simulink model "LTE_simulationslx"  (R2019a)
settings: Solver=ode45  StartTime=0.0  StopTime=0.003  RelTol=1e-3  EnableMultiTasking=on
undefined symbols (not defined in the file or in its folder): doppler, Iter, Len, Max, Variance
libraries: dspobslib x6, commsequence2 x6, commblkintrlv2 x6, dspindex x5, commcnvcod2 x4, commchan3 x2, commcrc2 x2, commdigbbndam3 x2, dspxfrm3 x2, commseqgen2 x2, commutil2 x2, commrandsrc3 x1
settings Model: Creator=Natalia  LastModifiedBy=Bill
settings DataIOCC: LimitDataPoints=on  SaveFormat=Array  SignalLoggingSaveFormat=ModelDataLogs  ReturnWorkspaceOutputs=off
settings OptimizationCC: ExpressionDepthLimit=2147483647  LifeSpan=inf
settings DebuggingCC: UnderspecifiedInitializationDetection=Classic  MergeDetectMultiDrivingBlocksExec=none  SolverPrmCheckMsg=warning  FcnCallInpInsideContextMsg=warning  StateNameClashWarn=warning  SFUnexpectedBacktrackingDiag=warning  SFNoUnconditionalDefaultTransitionDiag=warning  SFExecutionAtInitializationDiag=none  ArithmeticOperatorsInVariantConditions=warning
settings HardwareCC: ProdBitPerPointer=32  ProdBitPerSizeT=32  ProdBitPerPtrDiffT=32  ProdLargestAtomicFloat=None  ProdIntDivRoundTo=Undefined  ProdEndianess=Unspecified  ProdWordSize=32  ProdHWDeviceType=32-bit Generic
settings ModelReferenceCC: PropagateSignalLabelsOutOfModel=off
settings SFSimCC: SimUseLocalCustomCode=off  SimParseCustomCode=off
settings RTWCC: RTWUseLocalCustomCode=off
settings CodeAppCC: StateflowObjectComments=on
settings GRTTargetCC: TargetLangStandard=C89/C90 (ANSI)  GeneratePreprocessorConditionals=Disable all  CombineOutputUpdateFcns=off  GRTInterface=on
settings ConfigComp: CovMetricSettings=dw  CovHtmlReporting=on  CovSaveCumulativeToWorkspaceVar=on  CovSaveSingleToWorkspaceVar=on  CovExternalEMLEnable=off

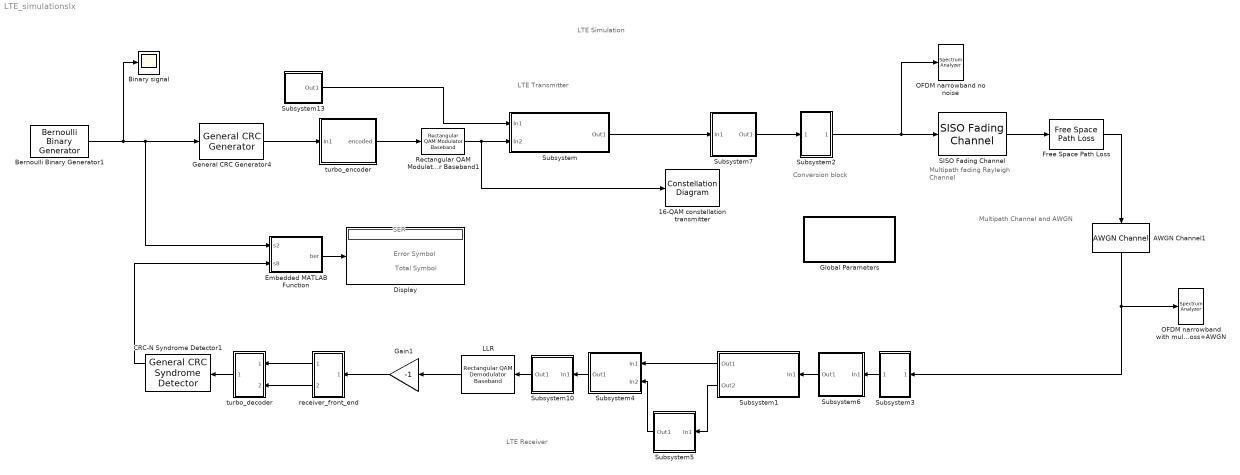
== system LTE_simulationslx ==
  note: SER
  note: Error Symbol
  note: Total Symbol
  note: LTE Simulation
  note: LTE Transmitter
  note: LTE Receiver
  note: Multipath Channel
      | and AWGN
  note: Conversion block
  note: Multipath fading Rayleigh Channel
  16-QAM constellation transmitter : ConstellationDiagram  Tag=ScatterPlot
  AWGN Channel1 : commchan3/AWGN Channel  InputProcessing=Columns as channels (frame based)  seed=32965  noiseMode="Signal to noise ratio  (Eb/No)"  EbNodB=12  EsNodB=1  SNRdB=2  bitsPerSym=1  Ps=30/(5.5e5*11/15*2.4)*1.08  Tsym=80e-6  variance=1
      settings: SourceProductName=Communications Toolbox
  Bernoulli Binary Generator1 : commrandsrc3/Bernoulli Binary Generator  ProbabilityOfZero=.5  SeedSource=Auto  Seed=0  SampleTime=1  SamplesPerFrame=20  OutputDataType=boolean  SimulateUsing=Code generation
      settings: SourceProductName=Communications Toolbox
  Binary signal : Scope
  CRC-N Syndrome Detector1 : commcrc2/General CRC Syndrome Detector  genPoly=[1 1 0 0 0 0 0 0 0 0 1 0 1 0 0 0 1 0 0 0 0 0 0 0 1]  iniStates=[0]  directMethod=off  reflectInputBytes=off  reflectChecksums=off  finalXOR=0  numChecksums=1
      settings: SourceProductName=Communications Toolbox  SourceProductBaseCode=CM
  Display : Display
  Embedded MATLAB Function : MATLAB Function  TreatAsAtomicUnit=on
  Free Space Path Loss : commrflib2/Free Space Path Loss  mode=Decibels  dB=10  d=0.100  fc=1920
      settings: SourceProductName=Communications Toolbox  SourceProductBaseCode=CM
  Gain1 : Gain  Gain=-1  SaturateOnIntegerOverflow=on  OutDataTypeStr=Inherit: Same as input  ParamDataTypeStr=Inherit: Same as input
  General CRC Generator4 : commcrc2/General CRC Generator  genPoly=[24,23,18,17,14,11,10,7,6,5,1,0]  iniStates=[0]  directMethod=off  reflectInputBytes=off  reflectChecksums=off  finalXOR=0  numChecksums=1
      settings: SourceProductName=Communications Toolbox  SourceProductBaseCode=CM
  Global Parameters : Subsystem  mask(Global Parameters){EbNodB=11, Len=44, Iter=5, Seed=54123}
      mask prompts: EbNodB "Eb/No in dB:"; Len "Block size:"; Iter "Number of iterations:"
      mask help: Load global parameters in MATLAB workspace.
      mask init:
      | turbo_code_punc_setup;
      mask Callback EbNodB: turbo_code_setup;
      mask Callback Len: turbo_code_setup
      mask Callback Iter: turbo_code_setup;
      mask Callback Seed: turbo_code_setup;
      mask Display: disp(['Eb/No ' num2str(EbNodB,'%3.1f') 'dB'  sprintf('\n') 'Block size   ' num2str(Len,'%7.0f')  sprintf('\n') 'Iterations   ' num2str(Iter,'%3.0f')   sprintf('\n') 'Seed   ' num2str(Seed,'%7.0f')])
  LLR : commdigbbndam3/Rectangular QAM Demodulator Baseband  M=16  OutType=Bit  DecType=Log-likelihood ratio  VarSource=Dialog  Variance=Variance  Dec=Gray  Mapping=[0:15]  PowType=Average Power  MinDist=2  AvgPow=0.5  PeakPow=1  Ph=0  outDtype1=double  outDtype2=double  derotateFactorWordLen=16  derotateFactorDataTypeStr=Inherit: Same word length as input  derotateFactorLastDataTypeStr=Inherit: Same word length as input  denormFactorWordLen=16  denormFactorDataTypeStr=Inherit: Same word length as input  denormFactorLastDataTypeStr=Inherit: Same word length as input  prodOutWordLen=32  prodOutOverflowMode=Wrap  prodOutRoundingMode=Floor  prodOutOvFlMode=off  prodOutOvFlModeLastStrValue=off  sumWordLen=32
      settings: SourceProductName=Communications Toolbox
  OFDM narrowband no noise : SpectrumAnalyzer
  OFDM narrowband with multipath fading +pathloss+AWGN : SpectrumAnalyzer
  Rectangular QAM Modulator Baseband1 : commdigbbndam3/Rectangular QAM Modulator Baseband  M=16  InType=Bit  Enc=Gray  Mapping=[0:15]  PowType=Average Power  MinDist=2  AvgPow=0.5  PeakPow=1  Ph=0  outDtype=double  outWordLen=16  outUDDataType=sfix(16)  outFracLenMode=Best precision  outFracLen=15  outDataTypeStr=double  outLastDataTypeStr=double
      settings: SourceProductName=Communications Toolbox
  SISO Fading Channel : commchan3/SISO Fading Channel  InheritSampleRate=on  SampleRate=1  PathDelays=[0 2e-6]  AveragePathGains=[0 -3]  NormalizePathGains=on  FadingDistribution=Rayleigh  KFactor=3  DirectPathDopplerShift=0  DirectPathInitialPhase=0  MaximumDopplerShift=40  DopplerSpectrum=doppler('Jakes')  ChannelInterpolationMethod=Polyphase  RandomStream=mt19937ar with seed  RandomNumGenerator=mt19937ar  Seed=73  PathGainsOutputPort=off  ChannelFilterDelayOutputPort=off  SimulateUsing=Interpreted execution  Visualization=Off  PathsForDopplerDisplay=1  SamplesToDisplay=25%
      settings: SourceProductName=Communications Toolbox
  Subsystem : Subsystem
      mask Display: disp('OFDM Baseband\nModulator\ndan\nAdd Cyclic Prefix')
  Subsystem1 : Subsystem
      mask Display: disp('OFDM Baseband\nDemodulator\ndan \nRemove Cyclic prefix')
  Subsystem10 : Subsystem
      mask Display: disp('Remove\nZero')
  Subsystem13 : Subsystem
      mask Display: disp('Training')
  Subsystem2 : Subsystem  Tag=Conversion block
      mask Display: disp('P/S')
  Subsystem3 : Subsystem
      mask Display: disp('S/P')
  Subsystem4 : Subsystem
      mask Display: disp('Channel\nCompensation')
  Subsystem5 : Subsystem
      mask Display: disp('Channel\nEstimator')
  Subsystem6 : Subsystem
      mask Display: disp('Training\nSeparation')
  Subsystem7 : Subsystem
      mask Display: disp('Training\nInsertion')
  receiver_front_end : Subsystem
  turbo_decoder : Subsystem
  turbo_encoder : Subsystem
  wires:
  receiver_front_end/1(Out1) -> turbo_decoder/1(In1)
  receiver_front_end/2(Out2) -> turbo_decoder/2(In2)
  turbo_encoder/1(encoded) -> Rectangular QAM Modulator Baseband1/1
  LLR/1 -> Gain1/1
  Gain1/1 -> receiver_front_end/1(In1)
  Subsystem13/1(Out1) -> Subsystem/1(In1)
  Subsystem/1(Out1) -> Subsystem7/1(In1)
  Subsystem7/1(Out1) -> Subsystem2/1(In1)
  Rectangular QAM Modulator Baseband1/1 -> 16-QAM constellation transmitter/1, Subsystem/2(In2)
  Subsystem1/1(Out1) -> Subsystem4/1(In1)
  Subsystem1/2(Out2) -> Subsystem5/1(In1)
  Subsystem5/1(Out1) -> Subsystem4/2(In2)
  Subsystem4/1(Out1) -> Subsystem10/1(In1)
  Subsystem6/1(Out1) -> Subsystem1/1(In1)
  Subsystem3/1(Out1) -> Subsystem6/1(In1)
  Subsystem10/1(Out1) -> LLR/1
  Subsystem2/1(Out1) -> OFDM narrowband no noise/1, SISO Fading Channel/1
  AWGN Channel1/1 -> OFDM narrowband with multipath fading +pathloss+AWGN/1, Subsystem3/1(In1)
  General CRC Generator4/1 -> turbo_encoder/1(In1)
  turbo_decoder/1(Out1) -> CRC-N Syndrome Detector1/1
  Embedded MATLAB Function/1(ber) -> Display/1
  CRC-N Syndrome Detector1/1 -> Embedded MATLAB Function/2(s8)
  Bernoulli Binary Generator1/1 -> Binary signal/1, Embedded MATLAB Function/1(s2), General CRC Generator4/1
  Free Space Path Loss/1 -> AWGN Channel1/1
  SISO Fading Channel/1 -> Free Space Path Loss/1

== system LTE_simulationslx/Global Parameters ==

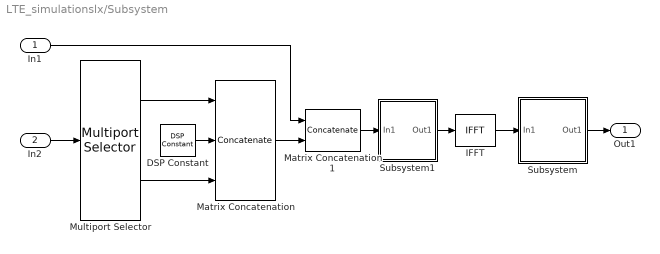
== system LTE_simulationslx/Subsystem ==
  In1 : Inport
  In2 : Inport  Port=2
  DSP Constant : dspobslib/DSP Constant  Value=0  SampleMode=Discrete  discreteOutput=Frame-based  continuousOutput=Sample-based  sampTime=16e-5/2  framePeriod=16e-5/2  dataType=Inherit from 'Constant value'  isSigned=on  wordLen=16  udDataType=sfix(16)  fracBitsMode=Best precision  numFracBits=15  InterpretAs1D=off  Ts=16e-5/2  FramebasedOutput=on
      settings: SourceProductName=DSP System Toolbox  SourceProductBaseCode=DS
  IFFT : dspxfrm3/IFFT  FFTImplementation=Auto  CompMethod=Table lookup  TableOpt=HYBRID  TableOptActive=Speed  BitRevOrder=off  cs_in=off  Normalize=on  InheritFFTLength=on  FFTLength=64  WrapInput=on  mode=Real  outSamplingMode=Frame based  roundingMode=Floor  overflowMode=off  firstCoeffDataTypeStr=Inherit: Same word length as input  firstCoeffLastDataTypeStr=Inherit: Same word length as input  outputMin=[]  outputMax=[]
      settings: SourceProductName=DSP System Toolbox
  Matrix Concatenation : Concatenate  NumInputs=3  Mode=Multidimensional array
  Matrix Concatenation1 : Concatenate  Mode=Multidimensional array  ConcatenateDimension=2
  Multiport Selector : dspindex/Multiport Selector  rowsOrCols=Rows  idxCellArray={1:11,12:22}  idxErrMode=Clip Index
  Subsystem : Subsystem
      mask Display: disp('Add\nCyclic Prefix')
  Subsystem1 : Subsystem
      mask Display: disp('Zero Pad')
  Out1 : Outport
  wires:
  IFFT/1 -> Subsystem/1(In1)
  Multiport Selector/1 -> Matrix Concatenation/1
  Multiport Selector/2 -> Matrix Concatenation/3
  DSP Constant/1 -> Matrix Concatenation/2
  Subsystem1/1(Out1) -> IFFT/1
  Subsystem/1(Out1) -> Out1/1
  In2/1 -> Multiport Selector/1
  Matrix Concatenation1/1 -> Subsystem1/1(In1)
  Matrix Concatenation/1 -> Matrix Concatenation1/2
  In1/1 -> Matrix Concatenation1/1

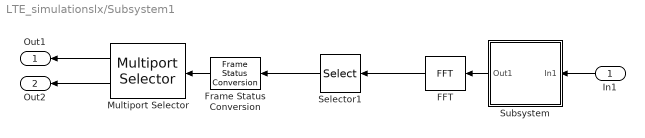
== system LTE_simulationslx/Subsystem1 ==
  In1 : Inport
  FFT : dspxfrm3/FFT  FFTImplementation=Auto  CompMethod=Table lookup  TableOpt=HYBRID  TableOptActive=Speed  BitRevOrder=off  Normalize=on  InheritFFTLength=on  FFTLength=64  WrapInput=on  roundingMode=Floor  overflowMode=off  firstCoeffDataTypeStr=Inherit: Same word length as input  firstCoeffLastDataTypeStr=Inherit: Same word length as input  outputMin=[]  outputMax=[]
  Frame Status Conversion : dspobslib/Frame Status Conversion  growRefPort=off  outframe=Frame-based
      settings: SourceProductName=DSP System Toolbox  SourceProductBaseCode=DS
  Multiport Selector : dspindex/Multiport Selector  rowsOrCols=Columns  idxCellArray={1,2}  idxErrMode=Clip Index
  Selector1 : Selector  NumberOfDimensions=2  InputPortWidth=64  IndexOptions=Index vector (dialog),Select all  Indices=[54:64,1:12],-1  OutputSizes=1
  Subsystem : Subsystem
      mask Display: disp('Remove\nCyclic Prefix')
  Out1 : Outport
  Out2 : Outport  Port=2
  wires:
  FFT/1 -> Selector1/1
  Selector1/1 -> Frame Status Conversion/1
  Subsystem/1(Out1) -> FFT/1
  In1/1 -> Subsystem/1(In1)
  Frame Status Conversion/1 -> Multiport Selector/1
  Multiport Selector/1 -> Out1/1
  Multiport Selector/2 -> Out2/1

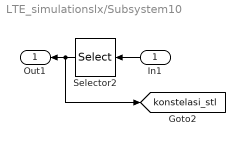
== system LTE_simulationslx/Subsystem10 ==
  In1 : Inport
  Selector2 : Selector  NumberOfDimensions=2  InputPortWidth=31  IndexOptions=Index vector (dialog),Select all  Indices=[1:11,13:23],-1  OutputSizes=1
  Out1 : Outport
  tag scope: konstelasi_stl=global
  wires:
  Selector2/1 -> Out1/1, [konstelasi_stl]
  In1/1 -> Selector2/1

== system LTE_simulationslx/Subsystem13 ==
  PN Sequence Generator : commseqgen2/PN Sequence Generator  poly=[1 0 0 0 0 1 1]  ini_sta=[0 0 0 0 0 1]  outBitMaskSource=Dialog parameter  shift=0  outVarSiz=off  maxOutSizeMode=Dialog parameter  maxOutSize=[10 1]  Ts=16e-5/2/23  frameBased=on  sampPerFrame=23  reset=off  bitPackedOutputs=off  outDataType=double  numPackedBits=8  bitPackDataSigned=off  bitPackedOutDType=double
      settings: SourceProductName=Communications Toolbox  SourceProductBaseCode=CM
  Unipolar to Bipolar Converter : commutil2/Unipolar to Bipolar Converter  M=2  polarity=Positive  dataType=Inherit via internal rule
      settings: SourceProductName=Communications Toolbox
  Out1 : Outport
  wires:
  PN Sequence Generator/1 -> Unipolar to Bipolar Converter/1
  Unipolar to Bipolar Converter/1 -> Out1/1

== system LTE_simulationslx/Subsystem2 ==
  In1 : Inport
  Unbuffer3 : Unbuffer
  Out1 : Outport
  wires:
  In1/1 -> Unbuffer3/1
  Unbuffer3/1 -> Out1/1

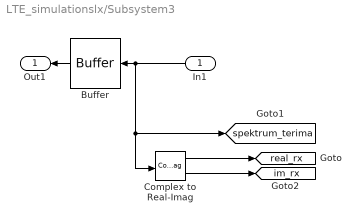
== system LTE_simulationslx/Subsystem3 ==
  In1 : Inport
  Buffer : Buffer  N=180
  Complex to Real-Imag : ComplexToRealImag
  Out1 : Outport
  tag scope: im_rx=global, real_rx=global, spektrum_terima=global
  wires:
  In1/1 -> Buffer/1, [spektrum_terima], Complex to Real-Imag/1
  Buffer/1 -> Out1/1
  Complex to Real-Imag/1 -> [real_rx]
  Complex to Real-Imag/2 -> [im_rx]

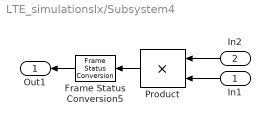
== system LTE_simulationslx/Subsystem4 ==
  In1 : Inport
  In2 : Inport  Port=2
  Frame Status Conversion5 : dspobslib/Frame Status Conversion  growRefPort=off  outframe=Frame-based
      settings: SourceProductName=DSP System Toolbox  SourceProductBaseCode=DS
  Product : Product  SaturateOnIntegerOverflow=on  OutDataTypeStr=Inherit: Same as first input
  Out1 : Outport
  wires:
  Product/1 -> Frame Status Conversion5/1
  Frame Status Conversion5/1 -> Out1/1
  In2/1 -> Product/1
  In1/1 -> Product/2

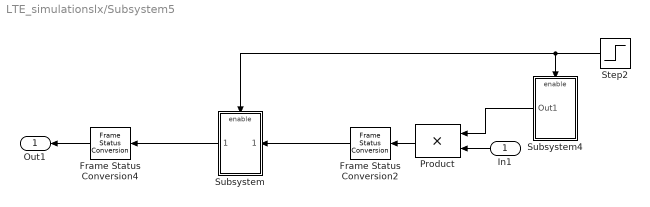
== system LTE_simulationslx/Subsystem5 ==
  In1 : Inport
  Frame Status Conversion2 : dspobslib/Frame Status Conversion  growRefPort=off  outframe=Frame-based
      settings: SourceProductName=DSP System Toolbox  SourceProductBaseCode=DS
  Frame Status Conversion4 : dspobslib/Frame Status Conversion  growRefPort=off  outframe=Frame-based
      settings: SourceProductName=DSP System Toolbox  SourceProductBaseCode=DS
  Product : Product  SaturateOnIntegerOverflow=on  OutDataTypeStr=Inherit: Same as first input
  Step2 : Step  Time=16e-5/2  SampleTime=16e-5/2
  Subsystem : Subsystem
  Subsystem4 : Subsystem  TreatAsAtomicUnit=on
  Out1 : Outport
  wires:
  Step2/1 -> Subsystem4/Enable, Subsystem/Enable
  Subsystem4/1(Out1) -> Product/1
  Product/1 -> Frame Status Conversion2/1
  Frame Status Conversion2/1 -> Subsystem/1(In1)
  Frame Status Conversion4/1 -> Out1/1
  In1/1 -> Product/2
  Subsystem/1(Out1) -> Frame Status Conversion4/1

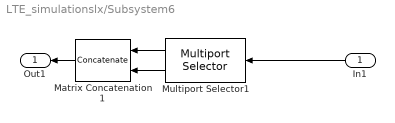
== system LTE_simulationslx/Subsystem6 ==
  In1 : Inport
  Matrix Concatenation1 : Concatenate  Mode=Multidimensional array  ConcatenateDimension=2
  Multiport Selector1 : dspindex/Multiport Selector  rowsOrCols=Rows  idxCellArray={91:180,1:90}  idxErrMode=Clip Index
  Out1 : Outport
  wires:
  Multiport Selector1/2 -> Matrix Concatenation1/2
  Multiport Selector1/1 -> Matrix Concatenation1/1
  In1/1 -> Multiport Selector1/1
  Matrix Concatenation1/1 -> Out1/1

== system LTE_simulationslx/Subsystem7 ==
  In1 : Inport
  Matrix Concatenation : Concatenate  Mode=Multidimensional array
  Multiport Selector : dspindex/Multiport Selector  rowsOrCols=Columns  idxCellArray={1,2}  idxErrMode=Clip Index
  Out1 : Outport
  wires:
  Multiport Selector/1 -> Matrix Concatenation/1
  Multiport Selector/2 -> Matrix Concatenation/2
  In1/1 -> Multiport Selector/1
  Matrix Concatenation/1 -> Out1/1

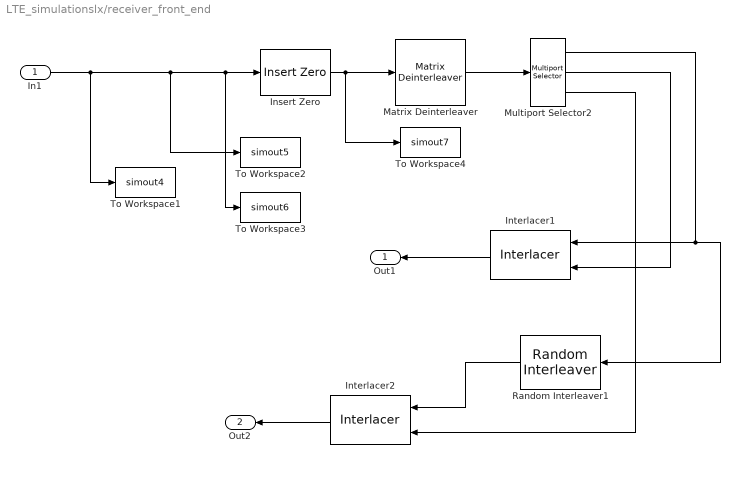
== system LTE_simulationslx/receiver_front_end ==
  In1 : Inport
  Insert Zero : commsequence2/Insert Zero  insertZeroVector=[1 1 0 1 0 1].'
      settings: SourceProductName=Communications Toolbox  SourceProductBaseCode=CM
  Interlacer1 : commsequence2/Interlacer
      settings: SourceProductName=Communications Toolbox  SourceProductBaseCode=CM
  Interlacer2 : commsequence2/Interlacer
      settings: SourceProductName=Communications Toolbox  SourceProductBaseCode=CM
  Matrix Deinterleaver : commblkintrlv2/Matrix Deinterleaver  Nrows=3  Ncols=44
      settings: SourceProductName=Communications Toolbox  SourceProductBaseCode=CM
  Multiport Selector2 : dspindex/Multiport Selector  rowsOrCols=Rows  idxCellArray={1:Len, Len+1:2*Len, 2*Len+1:3*Len}  idxErrMode=Clip Index
  Random Interleaver1 : commblkintrlv2/Random Interleaver  N=Len  seed=Seed
      settings: SourceProductName=Communications Toolbox  SourceProductBaseCode=CM
  To Workspace1 : ToWorkspace  VariableName=simout4  SampleTime=-1
  To Workspace2 : ToWorkspace  VariableName=simout5  SampleTime=-1
  To Workspace3 : ToWorkspace  VariableName=simout6  SampleTime=-1
  To Workspace4 : ToWorkspace  VariableName=simout7  SampleTime=-1
  Out1 : Outport
  Out2 : Outport  Port=2
  wires:
  Multiport Selector2/1 -> Interlacer1/1, Random Interleaver1/1
  Multiport Selector2/2 -> Interlacer1/2
  Random Interleaver1/1 -> Interlacer2/1
  Multiport Selector2/3 -> Interlacer2/2
  In1/1 -> To Workspace1/1, To Workspace2/1, Insert Zero/1, To Workspace3/1
  Interlacer1/1 -> Out1/1
  Interlacer2/1 -> Out2/1
  Matrix Deinterleaver/1 -> Multiport Selector2/1
  Insert Zero/1 -> Matrix Deinterleaver/1, To Workspace4/1

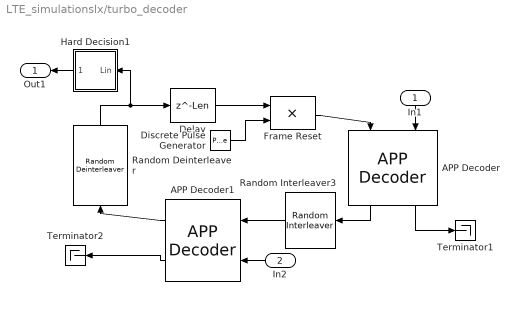
== system LTE_simulationslx/turbo_decoder ==
  In1 : Inport
  In2 : Inport  Port=2
  APP Decoder : commcnvcod2/APP Decoder  trellis=trellis  termMethod=Truncated  algorithm=Max*  maxStarNumScaleBits=3  disableLcOut=off
      settings: SourceProductName=Communications Toolbox  SourceProductBaseCode=CM
  APP Decoder1 : commcnvcod2/APP Decoder  trellis=trellis  termMethod=Truncated  algorithm=Max*  maxStarNumScaleBits=3  disableLcOut=off
      settings: SourceProductName=Communications Toolbox  SourceProductBaseCode=CM
  Delay : Delay  DelayLength=Len  InitialCondition=0  InputProcessing=Columns as channels (frame based)
  Discrete Pulse Generator : DiscretePulseGenerator  Period=Iter  PulseWidth=Iter-1  PhaseDelay=1
  Frame Reset : Product  SaturateOnIntegerOverflow=on  InputSameDT=on  OutDataTypeStr=Inherit: Same as first input
  Hard Decision1 : Subsystem  mask(Hard Decision){}
      mask help: Likelihood to binary transformation.
  Random Deinterleaver : commblkintrlv2/Random Deinterleaver  N=Len  seed=Seed
      settings: SourceProductName=Communications Toolbox  SourceProductBaseCode=CM
  Random Interleaver3 : commblkintrlv2/Random Interleaver  N=Len  seed=Seed
      settings: SourceProductName=Communications Toolbox  SourceProductBaseCode=CM
  Terminator1 : Terminator
  Terminator2 : Terminator
  Out1 : Outport
  wires:
  APP Decoder1/1 -> Random Deinterleaver/1
  APP Decoder/2 -> Terminator1/1
  APP Decoder1/2 -> Terminator2/1
  Random Deinterleaver/1 -> Delay/1, Hard Decision1/1(Lin)
  Random Interleaver3/1 -> APP Decoder1/1
  APP Decoder/1 -> Random Interleaver3/1
  Frame Reset/1 -> APP Decoder/1
  Delay/1 -> Frame Reset/1
  Discrete Pulse Generator/1 -> Frame Reset/2
  Hard Decision1/1(0/1) -> Out1/1
  In1/1 -> APP Decoder/2
  In2/1 -> APP Decoder1/2

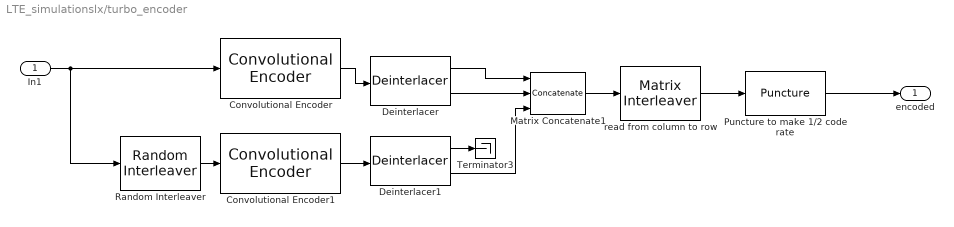
== system LTE_simulationslx/turbo_encoder ==
  In1 : Inport
  Convolutional Encoder : commcnvcod2/Convolutional Encoder  trellis=trellis  opMode=Continuous  DelayedResetAction=off  hasIniStPort=off  hasFinStPort=off  usePuncVector=off  punctureVector=[ 1 1 0 1 0 1]'  reset=Unused parameter value
      settings: SourceProductName=Communications Toolbox  SourceProductBaseCode=CM
  Convolutional Encoder1 : commcnvcod2/Convolutional Encoder  trellis=trellis  opMode=Truncated (reset every frame)  DelayedResetAction=off  hasIniStPort=off  hasFinStPort=off  usePuncVector=off  punctureVector=[ 1 1 0 1 0 1]'  reset=Unused parameter value
      settings: SourceProductName=Communications Toolbox  SourceProductBaseCode=CM
  Deinterlacer : commsequence2/Deinterlacer
      settings: SourceProductName=Communications Toolbox  SourceProductBaseCode=CM
  Deinterlacer1 : commsequence2/Deinterlacer
      settings: SourceProductName=Communications Toolbox  SourceProductBaseCode=CM
  Matrix Concatenate1 : Concatenate  NumInputs=3  Mode=Multidimensional array
  Puncture to make 1/2 code rate : commsequence2/Puncture  punctureVector=[1 1 0 1 0 1].'
      settings: SourceProductName=Communications Toolbox  SourceProductBaseCode=CM
  Random Interleaver : commblkintrlv2/Random Interleaver  N=Len  seed=Seed
      settings: SourceProductName=Communications Toolbox  SourceProductBaseCode=CM
  Terminator3 : Terminator
  read from column to row : commblkintrlv2/Matrix Interleaver  Nrows=3  Ncols=Len
      settings: SourceProductName=Communications Toolbox  SourceProductBaseCode=CM
  encoded : Outport
  wires:
  In1/1 -> Convolutional Encoder/1, Random Interleaver/1
  Puncture to make 1/2 code rate/1 -> encoded/1
  Random Interleaver/1 -> Convolutional Encoder1/1
  Convolutional Encoder/1 -> Deinterlacer/1
  Convolutional Encoder1/1 -> Deinterlacer1/1
  Deinterlacer1/1 -> Terminator3/1
  Deinterlacer/1 -> Matrix Concatenate1/1
  Deinterlacer1/2 -> Matrix Concatenate1/3
  read from column to row/1 -> Puncture to make 1/2 code rate/1
  Matrix Concatenate1/1 -> read from column to row/1
  Deinterlacer/2 -> Matrix Concatenate1/2

== system LTE_simulationslx/Subsystem/Subsystem ==
  In1 : Inport
  Selector3 : Selector  NumberOfDimensions=2  InputPortWidth=64  IndexOptions=Index vector (dialog),Select all  Indices=[39:64,1:64],-1  OutputSizes=1
  Out1 : Outport
  wires:
  Selector3/1 -> Out1/1
  In1/1 -> Selector3/1

== system LTE_simulationslx/Subsystem/Subsystem1 ==
  In1 : Inport
  Selector : Selector  NumberOfDimensions=2  InputPortWidth=64  IndexOptions=Index vector (dialog),Select all  Indices=[12:64,1:11],-1  OutputSizes=1
  Zero Pad : dspsigops/Pad  padAlong=Columns and rows  dimsToPad=1  valSrc=Specify via dialog  padVal=0  spec=Output size  padNumOutRowsSpecMethod=User-specified  numOutRows=64  padNumOutColsSpecMethod=User-specified  numOutCols=2  isVarDimsMode=off  padBeginning=0  padEnd=0  outSizeMode=User-specified  outSize=1  padSigAt=End  trunc_flag=None  roundingMode=Floor  overflowMode=off  truncOrWrapMode=Truncate  wrap_flag=None
      settings: SourceProductName=DSP System Toolbox  SourceProductBaseCode=DS
  Out1 : Outport
  wires:
  Zero Pad/1 -> Selector/1
  In1/1 -> Zero Pad/1
  Selector/1 -> Out1/1

== system LTE_simulationslx/Subsystem1/Subsystem ==
  In1 : Inport
  Selector4 : Selector  NumberOfDimensions=2  InputPortWidth=78  IndexOptions=Index vector (dialog),Select all  Indices=[27:90],-1  OutputSizes=1
  Out1 : Outport
  wires:
  Selector4/1 -> Out1/1
  In1/1 -> Selector4/1

== system LTE_simulationslx/Subsystem5/Subsystem ==
  In1 : Inport
  Enable : EnablePort
  Math Function : Math  Operator=reciprocal  SaturateOnIntegerOverflow=on
  Out1 : Outport
  wires:
  In1/1 -> Math Function/1
  Math Function/1 -> Out1/1

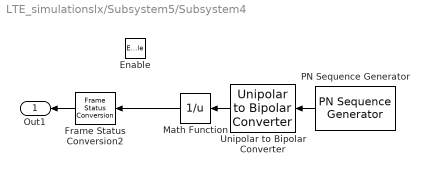
== system LTE_simulationslx/Subsystem5/Subsystem4 ==
  Enable : EnablePort
  Frame Status Conversion2 : dspobslib/Frame Status Conversion  growRefPort=off  outframe=Frame-based
      settings: SourceProductName=DSP System Toolbox  SourceProductBaseCode=DS
  Math Function : Math  Operator=reciprocal  SaturateOnIntegerOverflow=on
  PN Sequence Generator : commseqgen2/PN Sequence Generator  poly=[1 0 0 0 0 1 1]  ini_sta=[0 0 0 0 0 1]  outBitMaskSource=Dialog parameter  shift=0  outVarSiz=off  maxOutSizeMode=Dialog parameter  maxOutSize=[10 1]  Ts=16e-5/2/23  frameBased=on  sampPerFrame=23  reset=off  bitPackedOutputs=off  outDataType=double  numPackedBits=8  bitPackDataSigned=off  bitPackedOutDType=double
      settings: SourceProductName=Communications Toolbox  SourceProductBaseCode=CM
  Unipolar to Bipolar Converter : commutil2/Unipolar to Bipolar Converter  M=2  polarity=Positive  dataType=Inherit via internal rule
      settings: SourceProductName=Communications Toolbox
  Out1 : Outport
  wires:
  PN Sequence Generator/1 -> Unipolar to Bipolar Converter/1
  Frame Status Conversion2/1 -> Out1/1
  Math Function/1 -> Frame Status Conversion2/1
  Unipolar to Bipolar Converter/1 -> Math Function/1

== system LTE_simulationslx/turbo_decoder/Hard Decision1 ==
  Lin : Inport
  Constant : Constant  Value=0
  Relational Operator : RelationalOperator  RndMeth=Nearest  InputSameDT=on
  0/1 : Outport
  wires:
  Constant/1 -> Relational Operator/2
  Lin/1 -> Relational Operator/1
  Relational Operator/1 -> 0/1/1

== matlab function LTE_simulationslx/Embedded MATLAB Function ==
  data: s2 input; ber output; s8 input
function ber = fcn(s2,s8)
y=s2-s8;
z=0;
for i=1:20
    if y(i)~=0
        z=z+1;
    end
    
end
ber=z/(length(s2)*38);
